simulink model "Simulink_Full_Nonlinear_with_DOB"  (R2016a)
settings: Solver=VariableStepAuto  StartTime=0.0  StopTime=50  RelTol=1e-3
values from neighbouring files (symbols this model uses):
  a1 = 0.0135    [1TRAS_Nonlinear_Parameters.m]
  a2 = 0.02    [1TRAS_Nonlinear_Parameters.m]
  b1 = 0.0924    [1TRAS_Nonlinear_Parameters.m]
  B1phi = 0.1    [1TRAS_Nonlinear_Parameters.m]
  B1psi = 0.006    [1TRAS_Nonlinear_Parameters.m]
  b2 = 0.09    [1TRAS_Nonlinear_Parameters.m]
  B2psi = 0.001    [1TRAS_Nonlinear_Parameters.m]
  I1 = 0.068    [1TRAS_Nonlinear_Parameters.m]
  I2 = 0.02    [1TRAS_Nonlinear_Parameters.m]
  K1 = 1.1    [1TRAS_Nonlinear_Parameters.m]
  K2 = 0.8    [1TRAS_Nonlinear_Parameters.m]
  Kc = -0.2    [1TRAS_Nonlinear_Parameters.m]
  Kgy = 0.05    [1TRAS_Nonlinear_Parameters.m]
  Krm = lqr(A,B,Q,R)    [2LQG_For_TRAS_Pitch.m]
  Krt = lqr(A,B,Q,R)    [3LQG_for_TRAS_Yaw_angle.m]
  Mg = 0.32    [1TRAS_Nonlinear_Parameters.m]
  T0 = 3.5    [1TRAS_Nonlinear_Parameters.m]
  T10 = 1    [1TRAS_Nonlinear_Parameters.m]
  T11 = 1.1    [1TRAS_Nonlinear_Parameters.m]
  T20 = 1    [1TRAS_Nonlinear_Parameters.m]
  T21 = 1    [1TRAS_Nonlinear_Parameters.m]
  Tp = 2    [1TRAS_Nonlinear_Parameters.m]
undefined symbols (not defined in the file or in its folder): Akmain, Aktail, am, at, Bkmain, Bktail, bm, bt, Ckmain, Cktail, cm, ct, Dkmain, Dktail, Kem, Ket
libraries: cstblocks x1
settings Model: Creator=engrh  LastModifiedBy=engrh

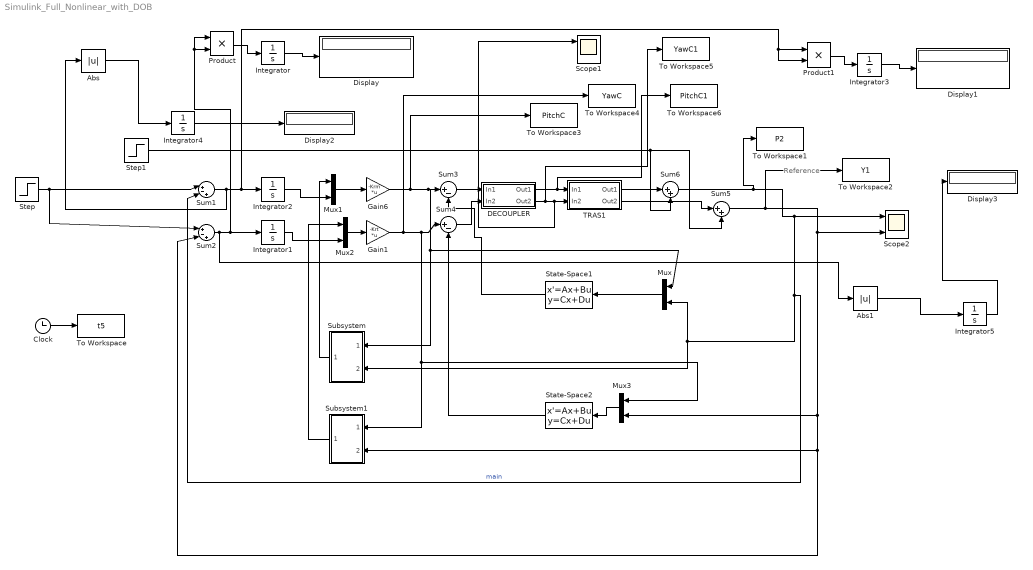
== system Simulink_Full_Nonlinear_with_DOB ==
  note: Reference
  Abs : Abs
  Abs1 : Abs
  Clock : Clock
  DECOUPLER : Subsystem
  Display{,1..3} (4 alike) : Display
  Gain1 : Gain  Gain=-Krt  Multiplication=Matrix(K*u)
  Gain6 : Gain  Gain=-Krm  Multiplication=Matrix(K*u)
  Integrator{,1..5} (6 alike) : Integrator
  Mux{,1..3} (4 alike) : Mux  Inputs=2
  Product : Product
  Product1 : Product
  Scope1 : Scope  NumInputPorts=2
  Scope2 : Scope  NumInputPorts=2
  State-Space1 : StateSpace  A=Akmain  B=Bkmain  C=Ckmain  D=Dkmain  X0=0
  State-Space2 : StateSpace  A=Aktail  B=Bktail  C=Cktail  D=Dktail  X0=0
  Step : Step  Time=0  SampleTime=0
  Step1 : Step  Time=30  After=0.5  SampleTime=0
  Subsystem : Subsystem
  Subsystem1 : Subsystem
  Sum1 : Sum  Inputs=|+-+
  Sum2 : Sum  Inputs=|+-+
  Sum3 : Sum  Inputs=|+-
  Sum4 : Sum  Inputs=|+-
  Sum5 : Sum  Inputs=|++
  Sum6 : Sum  Inputs=|++
  TRAS1 : Subsystem
  To Workspace : ToWorkspace  VariableName=t5  SampleTime=-1
  To Workspace1 : ToWorkspace  VariableName=P2  SampleTime=-1
  To Workspace2 : ToWorkspace  VariableName=Y1  SampleTime=-1
  To Workspace3 : ToWorkspace  VariableName=PitchC  SampleTime=-1
  To Workspace4 : ToWorkspace  VariableName=YawC  SampleTime=-1
  To Workspace5 : ToWorkspace  VariableName=YawC1  SampleTime=-1
  To Workspace6 : ToWorkspace  VariableName=PitchC1  SampleTime=-1
  wires:
  DECOUPLER/2(Out2) -> To Workspace5/1, Scope1/1, TRAS1/2(In2)
  DECOUPLER/1(Out1) -> To Workspace6/1, TRAS1/1(In1)
  Step/1 -> Sum2/1, Sum1/1
  Mux1/1 -> Gain6/1
  Integrator2/1 -> Mux1/2
  TRAS1/1(Out1) -> Sum6/1
  Sum6/1 -> To Workspace1/1, Scope2/1, Mux/2, Subsystem/2(In2), Sum1/2  "main"
  Subsystem/1(Out1) -> Mux1/1
  Mux2/1 -> Gain1/1
  Integrator1/1 -> Mux2/2
  Subsystem1/1(Out1) -> Mux2/1
  Sum5/1 -> To Workspace2/1, Scope2/2, Mux3/2, Sum2/2, Subsystem1/2(In2)
  Gain6/1 -> To Workspace3/1, Mux/1, Subsystem/1(In1), Sum3/1
  Sum3/1 -> DECOUPLER/1(In1)
  Step1/1 -> Sum6/2, Sum5/2
  Integrator/1 -> Display/1
  Product/1 -> Integrator/1
  Mux3/1 -> State-Space2/1
  State-Space2/1 -> Sum4/2
  Sum4/1 -> DECOUPLER/2(In2)
  Gain1/1 -> Sum4/1, Mux3/1, Subsystem1/1(In1), To Workspace4/1
  TRAS1/2(Out2) -> Sum5/1
  Clock/1 -> To Workspace/1
  State-Space1/1 -> Sum3/2
  Mux/1 -> State-Space1/1
  Integrator3/1 -> Display1/1
  Product1/1 -> Integrator3/1
  Sum1/1 -> Abs/1, Product1/2, Product1/1, Integrator2/1
  Integrator4/1 -> Display2/1
  Abs/1 -> Integrator4/1
  Sum2/1 -> Abs1/1, Product/2, Product/1, Integrator1/1
  Integrator5/1 -> Display3/1
  Abs1/1 -> Integrator5/1

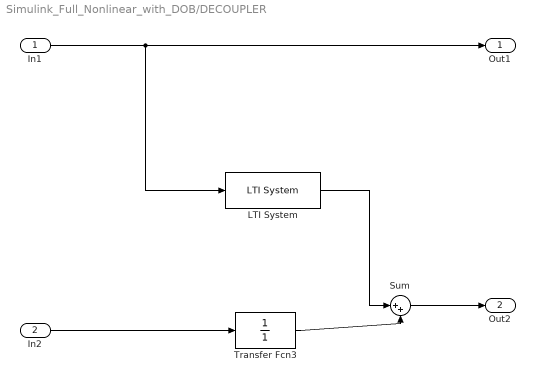
== system Simulink_Full_Nonlinear_with_DOB/DECOUPLER ==
  In1 : Inport
  In2 : Inport  Port=2
  LTI System : cstblocks/LTI System  sys=D21  IC=[]
  Sum : Sum  Inputs=|++
  Transfer Fcn3 : TransferFcn  Numerator=1  Denominator=1
  Out1 : Outport
  Out2 : Outport  Port=2
  wires:
  LTI System/1 -> Sum/1
  Transfer Fcn3/1 -> Sum/2
  Sum/1 -> Out2/1
  In1/1 -> Out1/1, LTI System/1
  In2/1 -> Transfer Fcn3/1

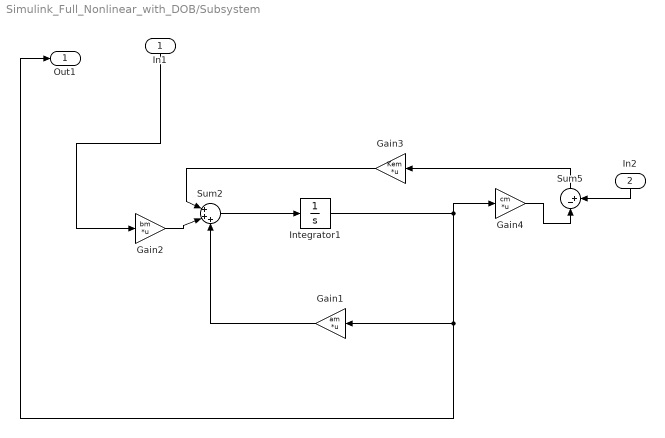
== system Simulink_Full_Nonlinear_with_DOB/Subsystem ==
  In1 : Inport
  In2 : Inport  Port=2
  Gain1 : Gain  Gain=am  Multiplication=Matrix(K*u)
  Gain2 : Gain  Gain=bm  Multiplication=Matrix(K*u)
  Gain3 : Gain  Gain=Kem  Multiplication=Matrix(K*u)
  Gain4 : Gain  Gain=cm  Multiplication=Matrix(K*u)
  Integrator1 : Integrator
  Sum2 : Sum  Inputs=|+++
  Sum5 : Sum  Inputs=|-+
  Out1 : Outport
  wires:
  Sum5/1 -> Gain3/1
  Gain3/1 -> Sum2/1
  Gain4/1 -> Sum5/1
  Gain1/1 -> Sum2/3
  Gain2/1 -> Sum2/2
  Sum2/1 -> Integrator1/1
  Integrator1/1 -> Out1/1, Gain1/1, Gain4/1
  In1/1 -> Gain2/1
  In2/1 -> Sum5/2

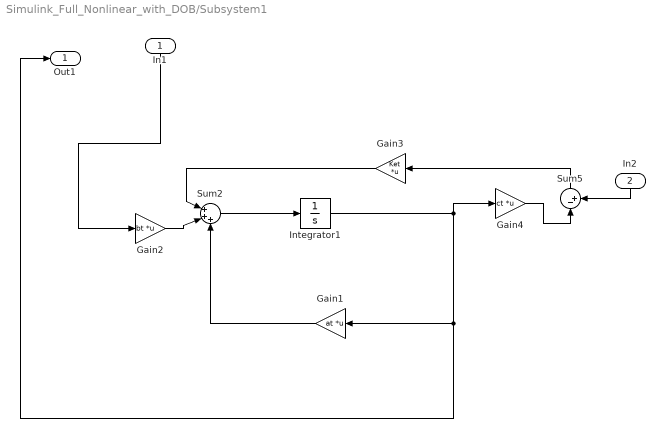
== system Simulink_Full_Nonlinear_with_DOB/Subsystem1 ==
  In1 : Inport
  In2 : Inport  Port=2
  Gain1 : Gain  Gain=at  Multiplication=Matrix(K*u)
  Gain2 : Gain  Gain=bt  Multiplication=Matrix(K*u)
  Gain3 : Gain  Gain=Ket  Multiplication=Matrix(K*u)
  Gain4 : Gain  Gain=ct  Multiplication=Matrix(K*u)
  Integrator1 : Integrator
  Sum2 : Sum  Inputs=|+++
  Sum5 : Sum  Inputs=|-+
  Out1 : Outport
  wires:
  Sum5/1 -> Gain3/1
  Gain3/1 -> Sum2/1
  Gain4/1 -> Sum5/1
  Gain1/1 -> Sum2/3
  Gain2/1 -> Sum2/2
  Sum2/1 -> Integrator1/1
  Integrator1/1 -> Out1/1, Gain1/1, Gain4/1
  In1/1 -> Gain2/1
  In2/1 -> Sum5/2

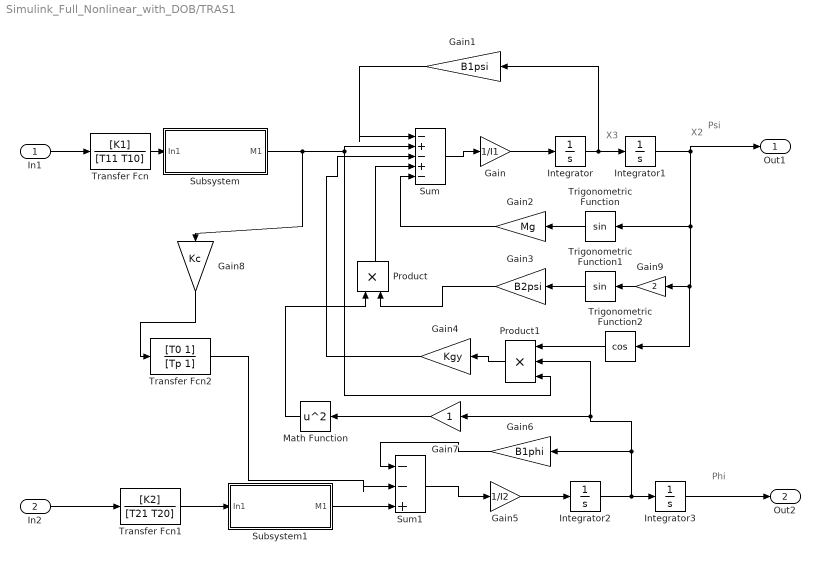
== system Simulink_Full_Nonlinear_with_DOB/TRAS1 ==
  note: Phi
  note: Psi
  note: X3
  note: X2
  In1 : Inport
  In2 : Inport  Port=2
  Gain : Gain  Gain=1/I1
  Gain1 : Gain  Gain=B1psi
  Gain2 : Gain  Gain=Mg
  Gain3 : Gain  Gain=B2psi
  Gain4 : Gain  Gain=Kgy
  Gain5 : Gain  Gain=1/I2
  Gain6 : Gain  Gain=B1phi
  Gain7 : Gain
  Gain8 : Gain  Gain=Kc
  Gain9 : Gain  Gain=2
  Integrator{,1..3} (4 alike) : Integrator
  Math Function : Math  Operator=square  SaturateOnIntegerOverflow=on
  Product : Product
  Product1 : Product  Inputs=3
  Subsystem : Subsystem
  Subsystem1 : Subsystem
  Sum : Sum  Inputs=|-+-+-
  Sum1 : Sum  Inputs=|--+
  Transfer Fcn : TransferFcn  Numerator=[K1]  Denominator=[T11 T10]
  Transfer Fcn1 : TransferFcn  Numerator=[K2]  Denominator=[T21 T20]
  Transfer Fcn2 : TransferFcn  Numerator=[T0 1]  Denominator=[Tp 1]
  Trigonometric Function : Trigonometry
  Trigonometric Function1 : Trigonometry
  Trigonometric Function2 : Trigonometry  Operator=cos
  Out1 : Outport
  Out2 : Outport  Port=2
  wires:
  In1/1 -> Transfer Fcn/1
  Transfer Fcn/1 -> Subsystem/1(In1)
  Sum/1 -> Gain/1
  Gain/1 -> Integrator/1
  Integrator/1 -> Gain1/1, Integrator1/1
  Integrator1/1 -> Gain9/1, Trigonometric Function2/1, Trigonometric Function/1, Out1/1
  Subsystem/1(M1) -> Gain8/1, Product1/3, Sum/2
  Gain1/1 -> Sum/1
  Gain2/1 -> Sum/5
  Gain3/1 -> Product/2
  Trigonometric Function/1 -> Gain2/1
  Trigonometric Function1/1 -> Gain3/1
  Product/1 -> Sum/4
  Trigonometric Function2/1 -> Product1/1
  Product1/1 -> Gain4/1
  Gain4/1 -> Sum/3
  In2/1 -> Transfer Fcn1/1
  Transfer Fcn1/1 -> Subsystem1/1(In1)
  Subsystem1/1(M1) -> Sum1/3
  Sum1/1 -> Gain5/1
  Gain5/1 -> Integrator2/1
  Integrator2/1 -> Gain7/1, Product1/2, Gain6/1, Integrator3/1
  Gain6/1 -> Sum1/1
  Gain7/1 -> Math Function/1
  Math Function/1 -> Product/1
  Gain8/1 -> Transfer Fcn2/1
  Transfer Fcn2/1 -> Sum1/2
  Integrator3/1 -> Out2/1
  Gain9/1 -> Trigonometric Function1/1

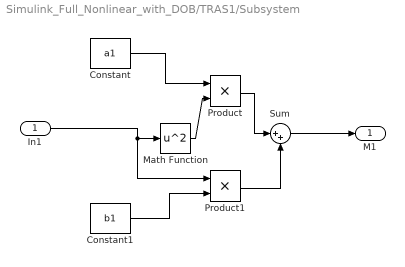
== system Simulink_Full_Nonlinear_with_DOB/TRAS1/Subsystem ==
  In1 : Inport
  Constant : Constant  Value=a1
  Constant1 : Constant  Value=b1
  Math Function : Math  Operator=square  SaturateOnIntegerOverflow=on
  Product : Product
  Product1 : Product
  Sum : Sum  Inputs=|++
  M1 : Outport
  wires:
  In1/1 -> Math Function/1, Product1/1
  Constant/1 -> Product/1
  Constant1/1 -> Product1/2
  Product/1 -> Sum/1
  Product1/1 -> Sum/2
  Sum/1 -> M1/1
  Math Function/1 -> Product/2

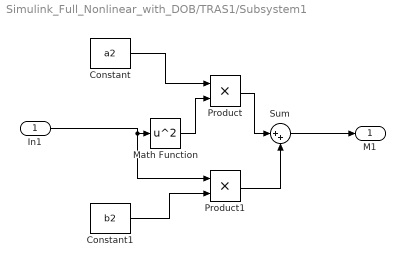
== system Simulink_Full_Nonlinear_with_DOB/TRAS1/Subsystem1 ==
  In1 : Inport
  Constant : Constant  Value=a2
  Constant1 : Constant  Value=b2
  Math Function : Math  Operator=square  SaturateOnIntegerOverflow=on
  Product : Product
  Product1 : Product
  Sum : Sum  Inputs=|++
  M1 : Outport
  wires:
  In1/1 -> Product1/1, Math Function/1
  Constant/1 -> Product/1
  Constant1/1 -> Product1/2
  Product/1 -> Sum/1
  Product1/1 -> Sum/2
  Sum/1 -> M1/1
  Math Function/1 -> Product/2
